simulink model "RailP_VDGradMon"  (R2016b)
settings: configuration reference "CodeGenConfigSet" (kept outside this file)
values from neighbouring files (symbols this model uses):
  RailP_dpMaxHyd_C = Calibration.Parameter    [init_RailP_VDGradMon.m]
  RailP_numdPDefDeb_C = Calibration.Parameter    [init_RailP_VDGradMon.m]
  RailP_numdPOKDeb_C = Calibration.Parameter    [init_RailP_VDGradMon.m]
  RailP_numGradExcdMax_C = Calibration.Parameter    [init_RailP_VDGradMon.m]
  RailP_tidPresRst_C = Calibration.Parameter    [init_RailP_VDGradMon.m]
undefined symbols (not defined in the file or in its folder): EngState_conv, RailP_VDGradMon_DT
libraries: CXLib x5
settings Model: Creator=Administrator  LastModifiedBy=Wei Liang
settings ConfigSetRef: SourceLocation=Base Workspace

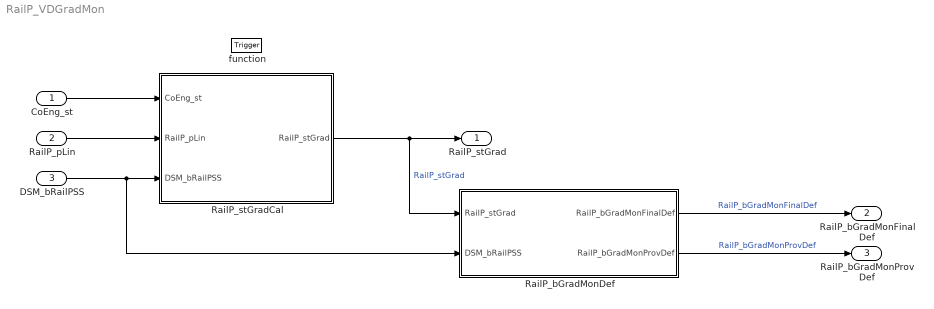
== system RailP_VDGradMon ==
  CoEng_st : Inport  Description=Engine coordinator state  OutDataTypeStr=Enum: EngState_conv
  RailP_pLin : Inport  Tag=bar  Description=Fuel pressure  Port=2  OutMin=0  OutMax=2500  OutDataTypeStr=RailPressure_bar
  DSM_bRailPSS : Inport  Description=Status of FId_RailPSS  Port=3  OutMin=0  OutMax=1  OutDataTypeStr=boolean
  function : TriggerPort  TriggerType=function-call  VariantControl=Variant
  RailP_bGradMonDef : Subsystem
  RailP_stGradCal : Subsystem
  RailP_stGrad : Outport  Description=Status of the gradient test  OutMin=0  OutMax=1  OutDataTypeStr=boolean
  RailP_bGradMonFinalDef : Outport  Description=Status of the final default for pressure gradient monitoring  Port=2  OutMin=0  OutMax=1  OutDataTypeStr=boolean
  RailP_bGradMonProvDef : Outport  Description="Status of the  provisional default for pressure gradient monitoring"  Port=3  OutMin=0  OutMax=1  OutDataTypeStr=boolean
  wires:
  DSM_bRailPSS/1 -> RailP_bGradMonDef/2(DSM_bRailPSS), RailP_stGradCal/3(DSM_bRailPSS)
  CoEng_st/1 -> RailP_stGradCal/1(CoEng_st)
  RailP_pLin/1 -> RailP_stGradCal/2(RailP_pLin)
  RailP_stGradCal/1(RailP_stGrad) -> RailP_stGrad/1, RailP_bGradMonDef/1(RailP_stGrad)  "RailP_stGrad"
  RailP_bGradMonDef/1(RailP_bGradMonFinalDef) -> RailP_bGradMonFinalDef/1  "RailP_bGradMonFinalDef"
  RailP_bGradMonDef/2(RailP_bGradMonProvDef) -> RailP_bGradMonProvDef/1  "RailP_bGradMonProvDef"

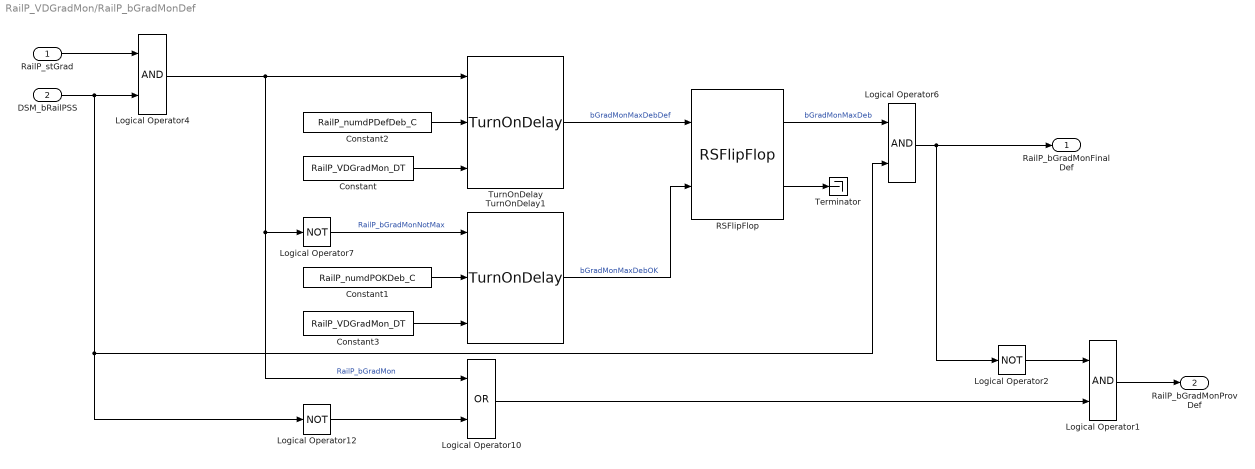
== system RailP_VDGradMon/RailP_bGradMonDef ==
  RailP_stGrad : Inport  Description=Engine operation status
  DSM_bRailPSS : Inport  Description=status of FId_RailPSS  Port=2  OutMin=0  OutMax=1  OutDataTypeStr=boolean
  Constant : Constant  Value=RailP_VDGradMon_DT  OutDataTypeStr=Inherit: Inherit via back propagation
  Constant1 : Constant  Value=RailP_numdPOKDeb_C
  Constant2 : Constant  Value=RailP_numdPDefDeb_C
  Constant3 : Constant  Value=RailP_VDGradMon_DT  OutDataTypeStr=Inherit: Inherit via back propagation
  Logical Operator1 : Logic  AllPortsSameDT=off  OutDataTypeStr=boolean
  Logical Operator10 : Logic  Operator=OR  AllPortsSameDT=off  OutDataTypeStr=boolean
  Logical Operator12 : Logic  Operator=NOT  AllPortsSameDT=off  OutDataTypeStr=boolean
  Logical Operator2 : Logic  Operator=NOT  AllPortsSameDT=off  OutDataTypeStr=boolean
  Logical Operator4 : Logic  AllPortsSameDT=off  OutDataTypeStr=boolean
  Logical Operator6 : Logic  AllPortsSameDT=off  OutDataTypeStr=boolean
  Logical Operator7 : Logic  Operator=NOT  AllPortsSameDT=off  OutDataTypeStr=boolean
  RSFlipFlop : CXLib/RSFlipFlop
  Terminator : Terminator
  TurnOnDelay : CXLib/TurnOnDelay
  TurnOnDelay1 : CXLib/TurnOnDelay
  RailP_bGradMonFinalDef : Outport  OutMin=0  OutMax=1  OutDataTypeStr=boolean
  RailP_bGradMonProvDef : Outport  Port=2  OutMin=0  OutMax=1  OutDataTypeStr=boolean
  wires:
  RailP_stGrad/1 -> Logical Operator4/1
  RSFlipFlop/1 -> Logical Operator6/1  "bGradMonMaxDeb"
  Logical Operator12/1 -> Logical Operator10/2
  Logical Operator6/1 -> Logical Operator2/1, RailP_bGradMonFinalDef/1
  Logical Operator4/1 -> Logical Operator10/1, Logical Operator7/1, TurnOnDelay/1  "RailP_bGradMon"
  TurnOnDelay1/1 -> RSFlipFlop/2  "bGradMonMaxDebOK"
  RSFlipFlop/2 -> Terminator/1
  Constant1/1 -> TurnOnDelay1/2
  Logical Operator7/1 -> TurnOnDelay1/1  "RailP_bGradMonNotMax"
  TurnOnDelay/1 -> RSFlipFlop/1  "bGradMonMaxDebDef"
  Constant2/1 -> TurnOnDelay/2
  Constant3/1 -> TurnOnDelay1/3
  Constant/1 -> TurnOnDelay/3
  DSM_bRailPSS/1 -> Logical Operator12/1, Logical Operator6/2, Logical Operator4/2
  Logical Operator10/1 -> Logical Operator1/2
  Logical Operator1/1 -> RailP_bGradMonProvDef/1
  Logical Operator2/1 -> Logical Operator1/1

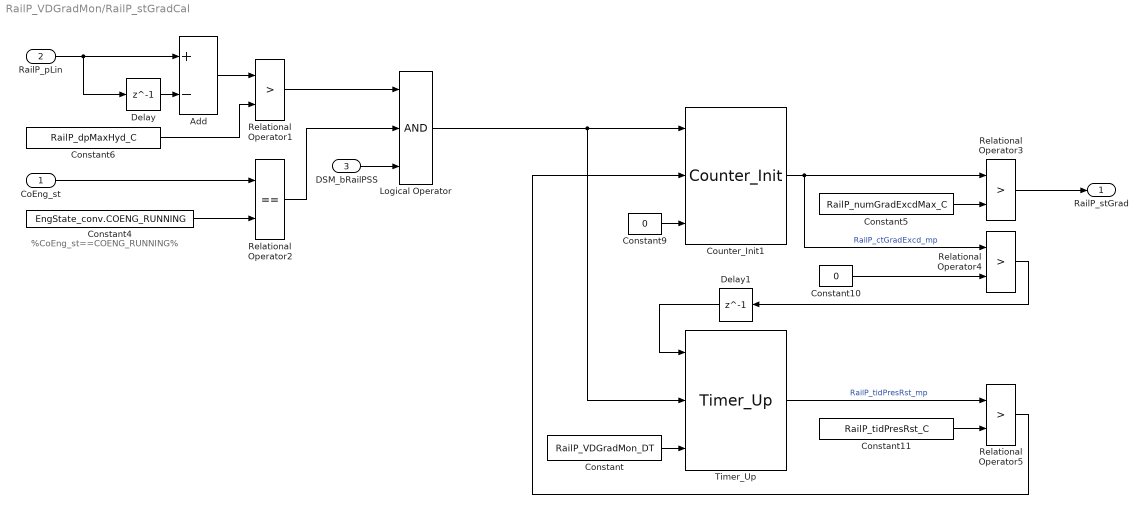
== system RailP_VDGradMon/RailP_stGradCal ==
  note: %CoEng_st==COENG_RUNNING%
  CoEng_st : Inport  Description=Engine operation status  OutDataTypeStr=Enum: EngState_conv
  RailP_pLin : Inport  Tag=bar  Description=Fuel pressure  Port=2  OutMin=0  OutMax=2500  OutDataTypeStr=RailPressure_bar
  DSM_bRailPSS : Inport  Description=status of FId_RailPSS  Port=3  OutMin=0  OutMax=1  OutDataTypeStr=boolean
  Add : Sum  Inputs=+-  OutDataTypeStr=Inherit: Inherit via back propagation  InputSameDT=on
  Constant : Constant  Value=RailP_VDGradMon_DT  OutDataTypeStr=Inherit: Inherit via back propagation
  Constant10 : Constant  Value=0  OutDataTypeStr=Inherit: Inherit via back propagation
  Constant11 : Constant  Value=RailP_tidPresRst_C
  Constant4 : Constant  Value=EngState_conv.COENG_RUNNING  OutDataTypeStr=Inherit: Inherit via back propagation
  Constant5 : Constant  Value=RailP_numGradExcdMax_C
  Constant6 : Constant  Value=RailP_dpMaxHyd_C
  Constant9 : Constant  Value=0  OutDataTypeStr=Inherit: Inherit via back propagation
  Counter_Init1 : CXLib/Counter_Init
  Delay : Delay  DelayLength=1  InitialCondition=0
  Delay1 : Delay  DelayLength=1  InitialCondition=0
  Logical Operator : Logic  Inputs=3  OutDataTypeStr=boolean
  Relational Operator{1,3..5} (4 alike) : RelationalOperator  Operator=>  OutDataTypeStr=boolean  RndMeth=Nearest  InputSameDT=on
  Relational Operator2 : RelationalOperator  Operator===  OutDataTypeStr=boolean  RndMeth=Nearest
  Timer_Up : CXLib/Timer_Up
  RailP_stGrad : Outport  OutMin=0  OutMax=1  OutDataTypeStr=boolean
  wires:
  Constant9/1 -> Counter_Init1/3
  Constant/1 -> Timer_Up/3
  DSM_bRailPSS/1 -> Logical Operator/3
  Relational Operator5/1 -> Counter_Init1/2
  Counter_Init1/1 -> Relational Operator3/1, Relational Operator4/1  "RailP_ctGradExcd_mp"
  Delay1/1 -> Timer_Up/1
  Constant11/1 -> Relational Operator5/2
  Timer_Up/1 -> Relational Operator5/1  "RailP_tidPresRst_mp"
  Relational Operator4/1 -> Delay1/1
  Constant10/1 -> Relational Operator4/2
  Relational Operator3/1 -> RailP_stGrad/1
  Constant5/1 -> Relational Operator3/2
  Relational Operator2/1 -> Logical Operator/2
  Relational Operator1/1 -> Logical Operator/1
  Constant4/1 -> Relational Operator2/2
  CoEng_st/1 -> Relational Operator2/1
  Constant6/1 -> Relational Operator1/2
  Add/1 -> Relational Operator1/1
  Delay/1 -> Add/2
  RailP_pLin/1 -> Delay/1, Add/1
  Logical Operator/1 -> Counter_Init1/1, Timer_Up/2
